simulink model "week1_prob6"  (R2020b)
settings: Solver=VariableStepAuto  StartTime=0.0  StopTime=10.0  RelTol=1e-3
settings Model: Creator=lalit  LastModifiedBy=lalit

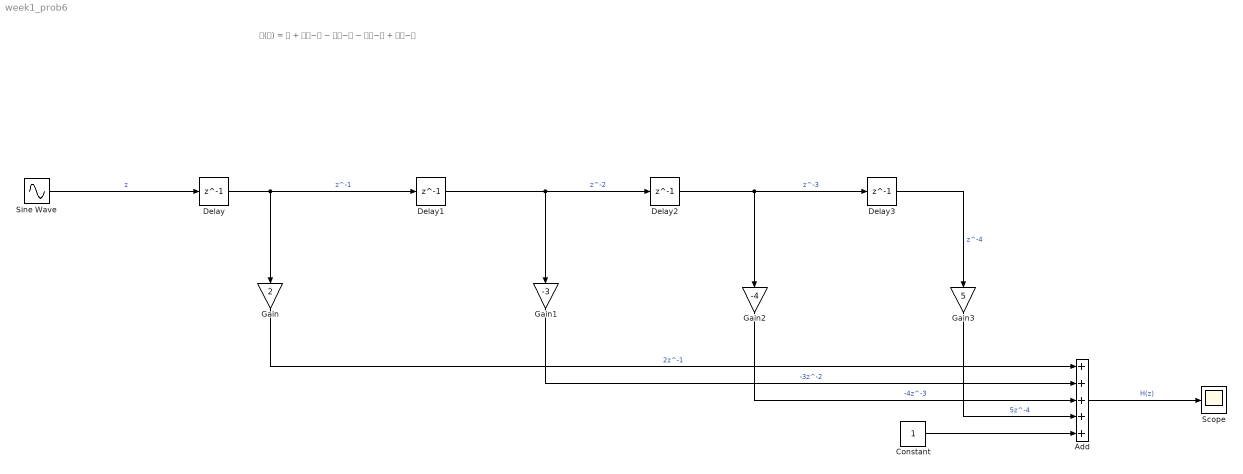
== system week1_prob6 ==
  note: 𝐇(𝐳) = 𝟏 + 𝟐𝐳−𝟏 − 𝟑𝐳−𝟐 − 𝟒𝐳−𝟑 + 𝟓𝐳−𝟒
  Add : Sum  Inputs=+++++
  Constant : Constant
  Delay{,1..3} (4 alike) : Delay  DelayLength=1
  Gain : Gain  Gain=2
  Gain1 : Gain  Gain=-3
  Gain2 : Gain  Gain=-4
  Gain3 : Gain  Gain=5
  Scope : Scope
  Sine Wave : Sin  SampleTime=0
  wires:
  Sine Wave/1 -> Delay/1  "z"
  Delay/1 -> Delay1/1, Gain/1  "z^-1"
  Delay1/1 -> Gain1/1, Delay2/1  "z^-2"
  Delay2/1 -> Gain2/1, Delay3/1  "z^-3"
  Delay3/1 -> Gain3/1  "z^-4"
  Gain/1 -> Add/1  "2z^-1"
  Gain1/1 -> Add/2  "-3z^-2"
  Gain2/1 -> Add/3  "-4z^-3"
  Gain3/1 -> Add/4  "5z^-4"
  Add/1 -> Scope/1  "H(z)"
  Constant/1 -> Add/5
